simulink model "buck_converter"  (R2025a)
settings: Solver=ode23tb  StartTime=0.0  StopTime=1  RelTol=1e-3
libraries: spsSeriesRLCBranchLib x3, spsVoltageMeasurementLib x2, spsCurrentMeasurementLib x1, spsDiodeLib x1, spsMosfetLib x1, spsPWMGeneratorDCDCLib x1, spsDCVoltageSourceLib x1, sps_lib x1
settings Model: Creator=SATYA  LastModifiedBy=SATYA

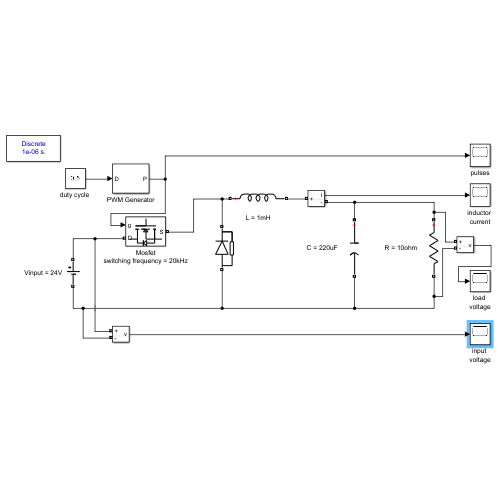
[thumbnail: Simulink's stored preview of the top-level diagram]
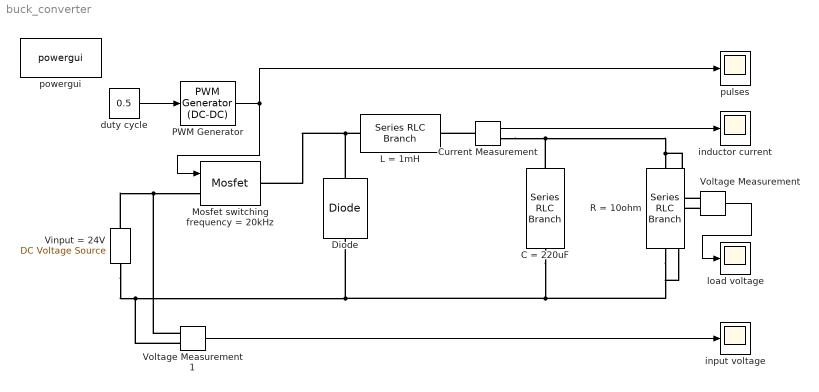
== system buck_converter ==
  C = 220uF : spsSeriesRLCBranchLib/Series RLC Branch  LConnTagsString=__new0  RConnTagsString=__new0  BranchType=C  Resistance=1  Inductance=1e-3  SetiL0=off  InitialCurrent=0  Capacitance=220e-6  Setx0=off  InitialVoltage=0  Measurements=Branch voltage
  Current Measurement : spsCurrentMeasurementLib/Current Measurement  PhasorSimulation=off  OutputType=Complex  PSBequivalent=0
  Diode : spsDiodeLib/Diode  Ron=0.001  Lon=0  Vf=0.8  IC=0  UseSnubber=0  Rs=500  Cs=250e-9  Measurements=off
  L = 1mH : spsSeriesRLCBranchLib/Series RLC Branch  LConnTagsString=__new0  RConnTagsString=__new0  BranchType=L  Resistance=1  Inductance=1e-3  SetiL0=off  InitialCurrent=0  Capacitance=1e-6  Setx0=off  InitialVoltage=0  Measurements=Branch current
  Mosfet switching frequency = 20kHz : spsMosfetLib/Mosfet  Ron=0.1  Lon=0  Rd=0.01  Vfd=0  IC=0  Rs=1e5  Cs=inf  Measurements=off
  PWM Generator : spsPWMGeneratorDCDCLib/PWM Generator (DC-DC)  Fsw=20000  Ts=0
  R = 10ohm : spsSeriesRLCBranchLib/Series RLC Branch  LConnTagsString=__new0  RConnTagsString=__new0  BranchType=R  Resistance=10  Inductance=1e-3  SetiL0=off  InitialCurrent=0  Capacitance=1e-6  Setx0=off  InitialVoltage=0  Measurements=Branch voltage
  Vinput = 24V : spsDCVoltageSourceLib/DC Voltage Source  Amplitude=24  Measurements=Voltage
  Voltage Measurement : spsVoltageMeasurementLib/Voltage Measurement  PhasorSimulation=off  OutputType=Complex  PSBequivalent=0
  Voltage Measurement1 : spsVoltageMeasurementLib/Voltage Measurement  PhasorSimulation=off  OutputType=Complex  PSBequivalent=0
  "duty cycle " : Constant  Value=0.5
  inductor current : Scope
      settings: Title=inductor current  ActiveDisplayYMinimum=-0.76065597016114539  ActiveDisplayYMaximum=6.7228941001119464  DataLoggingVariableName=ScopeData2
  input voltage : Scope
      settings: Title=input voltage  ActiveDisplayYMinimum=14  ActiveDisplayYMaximum=34
  load voltage : Scope
      settings: Title=voltage across load  ActiveDisplayYMinimum=-2.5347324351242082  ActiveDisplayYMaximum=22.836589516357854
  powergui : sps_lib/powergui  Priority=1  SimulationMode=Discrete  SampleTime=1e-6  frequency=60  Iterations=50  frequencyindice=0  Pbase=100e6  ErrMax=1e-4  UnitsV=kV  UnitsW=MW  buscounter=0  FunctionMessages=off  echomessages=off  EnableUseOfTLC=off  CurrentSourceSwitches=off  DisableSnubberDevices=off  DisableRonSwitches=off  DisableVfSwitches=off  DisplayEquations=off  AutomaticDiscreteSolvers=off  SolverType=Tustin/Backward Euler (TBE)  Interpol=off  ExternalGateDelay=off  methode=off  Ts=100  x0status=blocks  SPID=on  SwTol=0  HookPort=off  NonlinearTolerance=1e-4  nMaxIteration=100  ContinueOnMaxIteration=off  RestoreLinks=warning  ResistiveCurrentMeasurement=off  Frange=[0:2:500]  Ylog=off  Xlog=on  ShowGrid=off  save=off  variable=ZData  structure=0  ZoomFFT=off  StartTime=0.0  cycles=1  DisplayStyle=1  fundamental=60  FreqAxis=off  MaxFrequency=1000  frequencyindicesteady=1  RmsSteady=1  display=off
  pulses : Scope
      settings: ActiveDisplayYMinimum=-0.12499999999999997  ActiveDisplayYMaximum=1.125  DataLoggingVariableName=ScopeData3
  wires:
  PWM Generator/1 -> Mosfet switching frequency = 20kHz/1, pulses/1
  "duty cycle "/1 -> PWM Generator/1
  Voltage Measurement/1 -> load voltage/1
  Voltage Measurement1/1 -> input voltage/1
  Current Measurement/1 -> inductor current/1
  connections:
  Vinput = 24V/RConn1 -- Voltage Measurement1/LConn1 -- Mosfet switching frequency = 20kHz/LConn1
  L = 1mH/LConn1 -- Diode/RConn1 -- Mosfet switching frequency = 20kHz/RConn1
  C = 220uF/LConn1 -- Current Measurement/RConn1 -- Voltage Measurement/LConn1 -- R = 10ohm/LConn1
  Vinput = 24V/LConn1 -- Voltage Measurement1/LConn2 -- Voltage Measurement/LConn2 -- R = 10ohm/RConn1 -- C = 220uF/RConn1 -- Diode/LConn1
  Current Measurement/LConn1 -- L = 1mH/RConn1
